simulink model "quad_dynamics"  (R2026a)
settings: Solver=ode4  StopTime=50  FixedStep=0.001
InitFcn:
  | Quad_Constant
  | %Quad_Constant_Ferry
values from neighbouring files (symbols this model uses):
  Ax = 0.0    (= 0)    [Quad_Constant.m]    (also in Quad_Constant_Ferry.m = 0.1)
  Ay = 0.0    (= 0)    [Quad_Constant.m]    (also in Quad_Constant_Ferry.m = 0.1)
  Az = 0.0    (= 0)    [Quad_Constant.m]    (also in Quad_Constant_Ferry.m = 0.1)
  b = cT_rpm * rpm_to_rads_factor    (= 1.35552545536e-05)    [Quad_Constant.m]    (also in Quad_Constant_Ferry.m = 1.144e-08)
  d = cM_rpm * rpm_to_rads_factor    (= 2.66728015938e-07)    [Quad_Constant.m]    (also in Quad_Constant_Ferry.m = 9.94e-10)
  g = 9.8100    (= 9.81)    [Quad_Constant.m]    (also in Quad_Constant_Ferry.m)
  Ixx = 0.0095    [Quad_Constant.m]    (also in Quad_Constant_Ferry.m = 0.005)
  Iyy = 0.0095    [Quad_Constant.m]    (also in Quad_Constant_Ferry.m = 0.005)
  Izz = 0.0186    [Quad_Constant.m]    (also in Quad_Constant_Ferry.m = 0.01)
  Jr = 6.5e-07    [Quad_Constant.m]    (also in Quad_Constant_Ferry.m)
  l = 0.2223    [Quad_Constant.m]    (also in Quad_Constant_Ferry.m = 0.225)
  m = 1.0230    (= 1.023)    [Quad_Constant.m]    (also in Quad_Constant_Ferry.m = 0.284)
undefined symbols (not defined in the file or in its folder): fractalcoef
libraries: mspsensorlib x1
settings Model: Creator=Umesh  LastModifiedBy=choudharyumesh

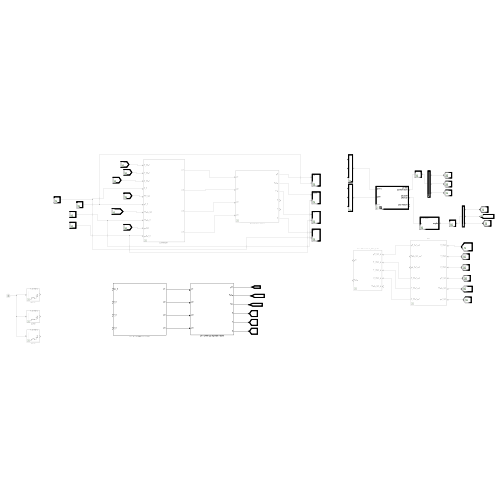
[thumbnail: Simulink's stored preview of the top-level diagram]
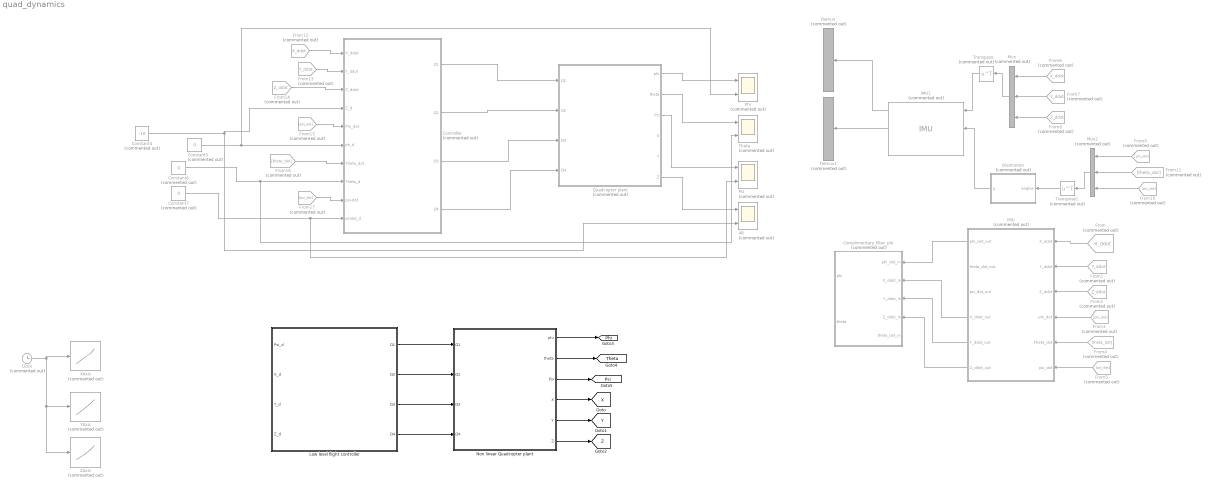
== system quad_dynamics ==
  Alt : Scope  Commented=on  NumInputPorts=2
      settings: ActiveDisplayYMinimum=-11.368140243902438  ActiveDisplayYMaximum=1.75685975609756
  Clock : Clock  Commented=on
  Complimentary_filter_phi : Subsystem  Commented=on
  Constant4 : Constant  Commented=on  Value=-10
  Constant5 : Constant  Commented=on  Value=0
  Constant6 : Constant  Commented=on  Value=0
  Constant7 : Constant  Commented=on  Value=0
  "Controller " : Subsystem  Commented=on
  Demux : Demux  Commented=on  Outputs=3
  Demux1 : Demux  Commented=on  Outputs=3
  From : From  Commented=on  GotoTag=X_ddot  TagVisibility=global
  From1 : From  Commented=on  GotoTag=Y_ddot  TagVisibility=global
  From10 : From  Commented=on  GotoTag=psi_dot  TagVisibility=global
  From11 : From  Commented=on  GotoTag=theta_dot  TagVisibility=global
  From12 : From  Commented=on  GotoTag=X_ddot  TagVisibility=global
  From13 : From  Commented=on  GotoTag=Y_ddot  TagVisibility=global
  From14 : From  Commented=on  GotoTag=Z_ddot  TagVisibility=global
  From15 : From  Commented=on  GotoTag=phi_dot  TagVisibility=global
  From16 : From  Commented=on  GotoTag=theta_dot  TagVisibility=global
  From17 : From  Commented=on  GotoTag=psi_dot  TagVisibility=global
  From2 : From  Commented=on  GotoTag=Z_ddot  TagVisibility=global
  From3 : From  Commented=on  GotoTag=phi_dot  TagVisibility=global
  From4 : From  Commented=on  GotoTag=theta_dot  TagVisibility=global
  From5 : From  Commented=on  GotoTag=psi_dot  TagVisibility=global
  From6 : From  Commented=on  GotoTag=X_ddot  TagVisibility=global
  From7 : From  Commented=on  GotoTag=Y_ddot  TagVisibility=global
  From8 : From  Commented=on  GotoTag=Z_ddot  TagVisibility=global
  From9 : From  Commented=on  GotoTag=phi_dot  TagVisibility=global
  IMU : Subsystem  Commented=on
  IMU1 : mspsensorlib/IMU  Commented=on  DispRefFrame=NED  TemperaturePort=off  Temperature=25  MagneticFieldPort=off  MagneticFieldNED=[ 27.5550, -2.4169, -16.0849 ]  MagneticFieldENU=[ -2.4169, 27.5550, 16.0849 ]  SeedDouble=67  SimulateUsing=Interpreted execution  AccelParamsMeasurementRange=Inf  AccelParamsResolution=0  AccelParamsConstantBias=[-2.755e-5, 1.565e-5, -9.942e-5]  AccelParamsAxesMisalignment=[ 100, 0, 0; 0, 100, 0; 0, 0, 100 ]  AccelParamsNoiseDensity=[ 0, 0, 0 ]  AccelParamsBiasInstability=[ 0, 0, 0 ]  AccelParamsBiasInstabilityNumerator=fractalcoef().Numerator  AccelParamsBiasInstabilityDenominator=fractalcoef().Denominator  AccelParamsRandomWalk=[ 0, 0, 0 ]  AccelParamsNoiseType=double-sided  AccelParamsTemperatureBias=[ 0, 0, 0 ]  AccelParamsTemperatureScaleFactor=[ 0, 0, 0 ]  GyroParamsMeasurementRange=Inf  GyroParamsResolution=0  GyroParamsConstantBias=[0.2001e-3, 0.2002e-3, 0.2004e-3]  GyroParamsAxesMisalignment=[ 100, 0, 0; 0, 100, 0; 0, 0, 100 ]  GyroParamsAccelerationBias=[ 0, 0, 0 ]  GyroParamsNoiseDensity=[ 0, 0, 0 ]  GyroParamsBiasInstability=[ 0, 0, 0 ]  GyroParamsBiasInstabilityNumerator=fractalcoef().Numerator  GyroParamsBiasInstabilityDenominator=fractalcoef().Denominator  GyroParamsRandomWalk=[ 0, 0, 0 ]  GyroParamsNoiseType=double-sided  GyroParamsTemperatureBias=[ 0, 0, 0 ]  GyroParamsTemperatureScaleFactor=[ 0, 0, 0 ]  MagParamsMeasurementRange=Inf  MagParamsResolution=0  MagParamsConstantBias=[-0.3223e-5, -0.1280e-5, 0.1589e-5]  MagParamsAxesMisalignment=[ 100, 0, 0; 0, 100, 0; 0, 0, 100 ]  MagParamsNoiseDensity=[ 0, 0, 0 ]  MagParamsBiasInstability=[ 0, 0, 0 ]  MagParamsBiasInstabilityNumerator=fractalcoef().Numerator  MagParamsBiasInstabilityDenominator=fractalcoef().Denominator  MagParamsRandomWalk=[ 0, 0, 0 ]  MagParamsNoiseType=double-sided  MagParamsTemperatureBias=[ 0, 0, 0 ]  MagParamsTemperatureScaleFactor=[ 0, 0, 0 ]
  Low level flight controller : Subsystem
  Mux : Mux  Commented=on  Inputs=3
  Mux2 : Mux  Commented=on  Inputs=3
  Non linear Quadcopter plant : Subsystem
  Oreintation : MATLAB Function  Commented=on  TreatAsAtomicUnit=on
  Phi : Scope  Commented=on  NumInputPorts=2
      settings: ActiveDisplayYMinimum=-5.7658911529616628  ActiveDisplayYMaximum=1.4877959493201969  DataLoggingVariableName=ScopeData2
  Psi : Scope  Commented=on  NumInputPorts=2
      settings: ActiveDisplayYMinimum=-3.9264406284982103  ActiveDisplayYMaximum=3.92682926955981
  Quadcopter plant : Subsystem  Commented=on
  Theta : Scope  Commented=on  NumInputPorts=2
      settings: ActiveDisplayYMinimum=-5.4636541903665821  ActiveDisplayYMaximum=1.4446192403780447  DataLoggingVariableName=ScopeData3
  Transpose : Math  Commented=on  Operator=transpose
  Transpose1 : Math  Commented=on  Operator=transpose
  XAxis : Lookup_n-D  Commented=on  NumberOfTableDimensions=1  BreakpointsForDimension1=[0, 5, 10, 15, 20, 25, 30]  Table=[0, 10, 0, -10, 0, 10, 0]  InterpMethod=Flat  InternalRulePriority=Speed  RndMeth=Simplest
  YAxis : Lookup_n-D  Commented=on  NumberOfTableDimensions=1  BreakpointsForDimension1=[0, 5, 10, 15, 20, 25, 30]  Table=[0, 0, 10, 0, -10, 0, 0]  InterpMethod=Flat  InternalRulePriority=Speed  RndMeth=Simplest
  ZAxis : Lookup_n-D  Commented=on  NumberOfTableDimensions=1  BreakpointsForDimension1=[0, 5, 10, 15, 20, 25, 30]  Table=[-3, -3, -3, -3, -3, -3, -3]  InterpMethod=Flat  InternalRulePriority=Speed  RndMeth=Simplest
  tag scope: Phi=global, Psi=global, Theta=global, X=global, Y=global, Z=global
  wires:
  From/1 -> IMU/1(X_ddot)
  From1/1 -> IMU/2(Y_ddot)
  From2/1 -> IMU/3(Z_ddot)
  From3/1 -> IMU/4(phi_dot)
  From4/1 -> IMU/5(Theta_dot)
  From5/1 -> IMU/6(psi_dot)
  IMU/1(phi_dot_out) -> Complimentary_filter_phi/1(phi_dot_in)
  IMU/4(X_ddot_out) -> Complimentary_filter_phi/2(X_ddot_in)
  IMU/5(Y_ddot_out) -> Complimentary_filter_phi/3(Y_ddot_in)
  IMU/6(Z_ddot_out) -> Complimentary_filter_phi/4(Z_ddot_in)
  From6/1 -> Mux/1
  From7/1 -> Mux/2
  From8/1 -> Mux/3
  Mux/1 -> Transpose/1
  From9/1 -> Mux2/1
  From10/1 -> Mux2/3
  From11/1 -> Mux2/2
  Mux2/1 -> Transpose1/1
  "Controller "/1(Ω1) -> Quadcopter plant/1(Ω1)
  "Controller "/2(Ω2) -> Quadcopter plant/2(Ω2)
  "Controller "/3(Ω3) -> Quadcopter plant/3(Ω3)
  "Controller "/4(Ω4) -> Quadcopter plant/4(Ω4)
  IMU1/2 -> Demux1/1
  IMU1/1 -> Demux/1
  Transpose/1 -> IMU1/1
  Transpose1/1 -> Oreintation/1(angles)
  Oreintation/1(q) -> IMU1/2
  From17/1 -> "Controller "/9(psi-dot)
  From16/1 -> "Controller "/7(Theta_dot)
  From15/1 -> "Controller "/5(Phi_dot)
  From12/1 -> "Controller "/1(X_ddot)
  From13/1 -> "Controller "/2(Y_ddot)
  From14/1 -> "Controller "/3(Z_ddot)
  Constant4/1 -> "Controller "/4(Z_d), Alt/2
  Constant5/1 -> Phi/2, "Controller "/6(ph_d)
  Constant6/1 -> Theta/2, "Controller "/8(Theta_d)
  Constant7/1 -> Psi/2, "Controller "/10(psidot_d)
  Quadcopter plant/6(Z) -> Alt/1
  Quadcopter plant/1(phi) -> Phi/1
  Quadcopter plant/2(theta) -> Theta/1
  Quadcopter plant/3(Psi) -> Psi/1
  Non linear Quadcopter plant/2(theta) -> [Theta]
  Non linear Quadcopter plant/3(Psi) -> [Psi]
  Non linear Quadcopter plant/4(X) -> [X]
  Non linear Quadcopter plant/5(Y) -> [Y]
  Non linear Quadcopter plant/6(Z) -> [Z]
  Low level flight controller/1(Ω1) -> Non linear Quadcopter plant/1(Ω1)
  Low level flight controller/2(Ω2) -> Non linear Quadcopter plant/2(Ω2)
  Low level flight controller/3(Ω3) -> Non linear Quadcopter plant/3(Ω3)
  Low level flight controller/4(Ω4) -> Non linear Quadcopter plant/4(Ω4)
  Clock/1 -> ZAxis/1, YAxis/1, XAxis/1
  Non linear Quadcopter plant/1(phi) -> [Phi]

== system quad_dynamics/Complimentary_filter_phi ==
  phi_dot_in : Inport
  X_ddot_in : Inport  Port=2
  Y_ddot_in : Inport  Port=3
  Z_ddot_in : Inport  Port=4
  theta_dot_in : Inport  Port=5
  High pass filter : TransferFcn  Numerator=[2 0]  Denominator=[2 1]
  High pass filter1 : TransferFcn  Numerator=[2 0]  Denominator=[2 1]
  Integrator : Integrator
  Integrator1 : Integrator
  Low pass filter : TransferFcn  Denominator=[2 1]
  MATLAB Function : MATLAB Function  TreatAsAtomicUnit=on
  Sum : Sum
  Sum1 : Sum
  phi : Outport
  theta : Outport  Port=2
  wires:
  X_ddot_in/1 -> MATLAB Function/1(X_ddot_in)
  Y_ddot_in/1 -> MATLAB Function/2(Y_ddot_in)
  Z_ddot_in/1 -> MATLAB Function/3(Z_ddot_in)
  MATLAB Function/1(Phi) -> Low pass filter/1
  phi_dot_in/1 -> Integrator/1
  Integrator/1 -> High pass filter/1
  Low pass filter/1 -> Sum/1
  High pass filter/1 -> Sum/2
  Sum/1 -> phi/1
  theta_dot_in/1 -> Integrator1/1
  Integrator1/1 -> High pass filter1/1
  High pass filter1/1 -> Sum1/2
  MATLAB Function/2(Theta) -> Sum1/1
  Sum1/1 -> theta/1

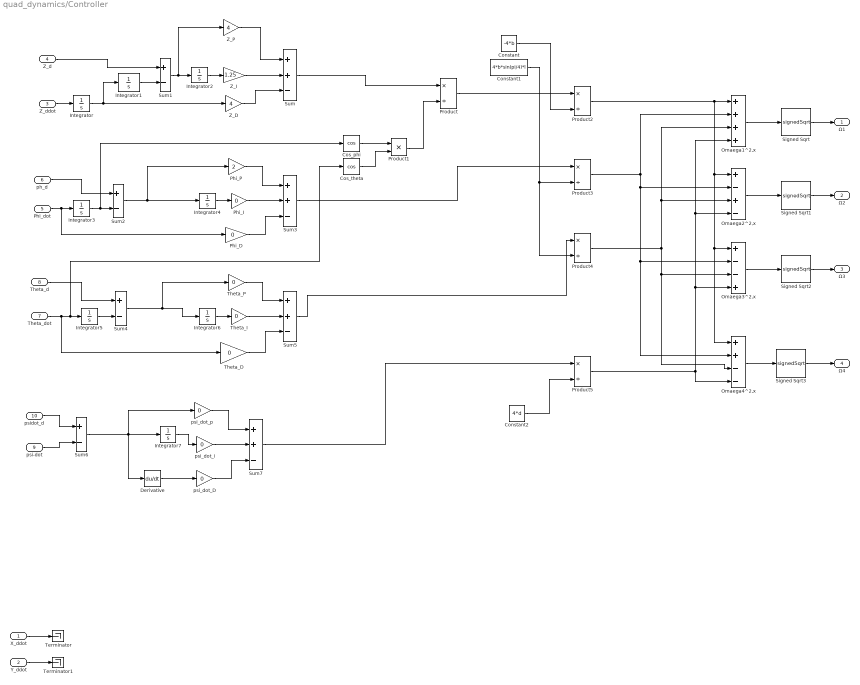
== system quad_dynamics/Controller  ==
  X_ddot : Inport
  Y_ddot : Inport  Port=2
  Z_ddot : Inport  Port=3
  Z_d : Inport  Port=4
  Phi_dot : Inport  Port=5
  ph_d : Inport  Port=6
  Theta_dot : Inport  Port=7
  Theta_d : Inport  Port=8
  psi-dot : Inport  Port=9
  psidot_d : Inport  Port=10
  Constant : Constant  Value=-4*b
  Constant1 : Constant  Value=4*b*sin(pi/4)*l
  Constant2 : Constant  Value=4*d
  Cos_phi : Trigonometry  Operator=cos
  Cos_theta : Trigonometry  Operator=cos
  Derivative : Derivative
  Integrator{,4,6..7} (4 alike) : Integrator
  Integrator1 : Integrator  UpperSaturationLimit=pi  LowerSaturationLimit=-pi
  Integrator2 : Integrator  LimitOutput=on  UpperSaturationLimit=5  LowerSaturationLimit=-5
  Integrator3 : Integrator  UpperSaturationLimit=pi  LowerSaturationLimit=-pi  WrapState=on
  Integrator5 : Integrator  UpperSaturationLimit=pi  LowerSaturationLimit=-pi  WrapState=on
  Omaega1^2,x : Sum  Inputs=++++
  Omaega2^2,x : Sum  Inputs=+-+-
  Omaega3^2,x : Sum  Inputs=+--+
  Omaega4^2,x : Sum  Inputs=++--
  Phi_D : Gain  Gain=0
  Phi_I : Gain  Gain=0
  Phi_P : Gain  Gain=2
  Product{,2..5} (5 alike) : Product  Inputs=*/
  Product1 : Product
  Signed Sqrt{,1..3} (4 alike) : Sqrt  Operator=signedSqrt
  Sum{,3,5,7} (4 alike) : Sum  Inputs=++-
  Sum{1..2,4,6} (4 alike) : Sum  Inputs=+-
  Terminator : Terminator
  Terminator1 : Terminator
  Theta_D : Gain  Gain=0
  Theta_I : Gain  Gain=0
  Theta_P : Gain  Gain=0
  Z_D : Gain  Gain=4
  Z_I : Gain  Gain=1.25
  Z_P : Gain  Gain=4
  psi_dot_D : Gain  Gain=0
  psi_dot_i : Gain  Gain=0
  psi_dot_p : Gain  Gain=0
  Ω1 : Outport
  Ω2 : Outport  Port=2
  Ω3 : Outport  Port=3
  Ω4 : Outport  Port=4
  wires:
  Z_ddot/1 -> Integrator/1
  Integrator/1 -> Z_D/1, Integrator1/1
  Integrator1/1 -> Sum1/2
  Z_d/1 -> Sum1/1
  Z_D/1 -> Sum/3
  Integrator2/1 -> Z_I/1
  Z_I/1 -> Sum/2
  Z_P/1 -> Sum/1
  Sum1/1 -> Z_P/1, Integrator2/1
  Phi_dot/1 -> Phi_D/1, Integrator3/1
  Integrator3/1 -> Cos_phi/1, Sum2/2
  ph_d/1 -> Sum2/1
  Phi_D/1 -> Sum3/3
  Integrator4/1 -> Phi_I/1
  Sum2/1 -> Phi_P/1, Integrator4/1
  Phi_I/1 -> Sum3/2
  Phi_P/1 -> Sum3/1
  Integrator5/1 -> Sum4/2
  Theta_d/1 -> Sum4/1
  Theta_P/1 -> Sum5/1
  Theta_dot/1 -> Theta_D/1, Cos_theta/1, Integrator5/1
  Theta_D/1 -> Sum5/3
  Theta_I/1 -> Sum5/2
  Integrator6/1 -> Theta_I/1
  Sum4/1 -> Theta_P/1, Integrator6/1
  psidot_d/1 -> Sum6/1
  psi_dot_i/1 -> Sum7/2
  Integrator7/1 -> psi_dot_i/1
  psi_dot_D/1 -> Sum7/3
  psi_dot_p/1 -> Sum7/1
  Sum6/1 -> Derivative/1, Integrator7/1, psi_dot_p/1
  Derivative/1 -> psi_dot_D/1
  Sum/1 -> Product/1
  Cos_phi/1 -> Product1/1
  Cos_theta/1 -> Product1/2
  Product1/1 -> Product/2
  Product/1 -> Product2/1
  Constant/1 -> Product2/2
  Constant1/1 -> Product4/2, Product3/2
  Sum3/1 -> Product3/1
  Sum5/1 -> Product4/1
  Sum7/1 -> Product5/1
  Constant2/1 -> Product5/2
  Omaega1^2,x/1 -> Signed Sqrt/1
  Signed Sqrt/1 -> Ω1/1
  Product2/1 -> Omaega4^2,x/1, Omaega3^2,x/1, Omaega2^2,x/1, Omaega1^2,x/1
  Product3/1 -> Omaega4^2,x/2, Omaega3^2,x/2, Omaega2^2,x/2, Omaega1^2,x/2
  Product4/1 -> Omaega3^2,x/3, Omaega4^2,x/3, Omaega2^2,x/3, Omaega1^2,x/3
  Product5/1 -> Omaega3^2,x/4, Omaega2^2,x/4, Omaega1^2,x/4, Omaega4^2,x/4
  Omaega2^2,x/1 -> Signed Sqrt1/1
  Signed Sqrt1/1 -> Ω2/1
  Omaega3^2,x/1 -> Signed Sqrt2/1
  Signed Sqrt2/1 -> Ω3/1
  Omaega4^2,x/1 -> Signed Sqrt3/1
  Signed Sqrt3/1 -> Ω4/1
  X_ddot/1 -> Terminator/1
  Y_ddot/1 -> Terminator1/1
  psi-dot/1 -> Sum6/2

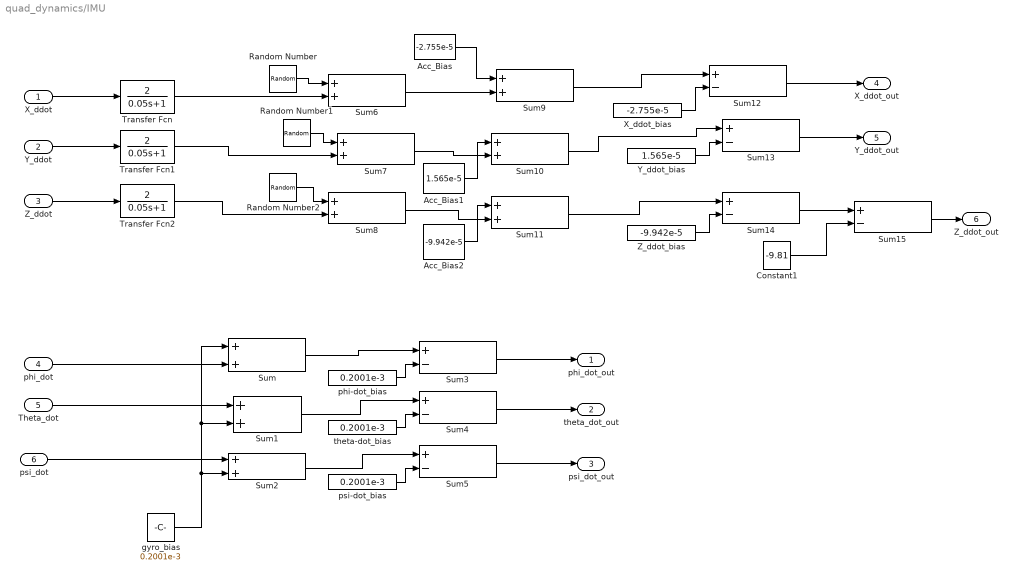
== system quad_dynamics/IMU ==
  X_ddot : Inport
  Y_ddot : Inport  Port=2
  Z_ddot : Inport  Port=3
  phi_dot : Inport  Port=4
  Theta_dot : Inport  Port=5
  psi_dot : Inport  Port=6
  Acc_Bias : Constant  Value=-2.755e-5
  Acc_Bias1 : Constant  Value=1.565e-5
  Acc_Bias2 : Constant  Value=-9.942e-5
  Constant1 : Constant  Value=-9.81
  Random Number : RandomNumber  Variance=0  Seed=1  SampleTime=0.01
  Random Number1 : RandomNumber  Variance=0  Seed=1  SampleTime=0.01
  Random Number2 : RandomNumber  Variance=0  Seed=1  SampleTime=0.01
  Sum{,1..2,6..11} (9 alike) : Sum
  Sum{3..5,12..15} (7 alike) : Sum  Inputs=+-
  Transfer Fcn : TransferFcn  Numerator=[2]  Denominator=[0.05 1]
  Transfer Fcn1 : TransferFcn  Numerator=[2]  Denominator=[0.05 1]
  Transfer Fcn2 : TransferFcn  Numerator=[2]  Denominator=[0.05 1]
  X_ddot_bias : Constant  Value=-2.755e-5
  Y_ddot_bias : Constant  Value=1.565e-5
  Z_ddot_bias : Constant  Value=-9.942e-5
  gyro_bias : Constant  Value=0.2001e-3
  phi-dot_bias : Constant  Value=0.2001e-3
  psi-dot_bias : Constant  Value=0.2001e-3
  theta-dot_bias : Constant  Value=0.2001e-3
  phi_dot_out : Outport
  theta_dot_out : Outport  Port=2
  psi_dot_out : Outport  Port=3
  X_ddot_out : Outport  Port=4
  Y_ddot_out : Outport  Port=5
  Z_ddot_out : Outport  Port=6
  wires:
  gyro_bias/1 -> Sum/1, Sum1/2, Sum2/2
  phi_dot/1 -> Sum/2
  Theta_dot/1 -> Sum1/1
  psi_dot/1 -> Sum2/1
  Sum/1 -> Sum3/1
  Sum1/1 -> Sum4/1
  Sum2/1 -> Sum5/1
  phi-dot_bias/1 -> Sum3/2
  theta-dot_bias/1 -> Sum4/2
  psi-dot_bias/1 -> Sum5/2
  Sum3/1 -> phi_dot_out/1
  Sum4/1 -> theta_dot_out/1
  Sum5/1 -> psi_dot_out/1
  Random Number2/1 -> Sum8/1
  Random Number1/1 -> Sum7/1
  Random Number/1 -> Sum6/1
  Sum6/1 -> Sum9/2
  Sum7/1 -> Sum10/2
  Sum8/1 -> Sum11/2
  Acc_Bias/1 -> Sum9/1
  Sum9/1 -> Sum12/1
  X_ddot_bias/1 -> Sum12/2
  Y_ddot_bias/1 -> Sum13/2
  Z_ddot_bias/1 -> Sum14/2
  Sum10/1 -> Sum13/1
  Sum11/1 -> Sum14/1
  Sum14/1 -> Sum15/1
  Constant1/1 -> Sum15/2
  Sum15/1 -> Z_ddot_out/1
  Sum13/1 -> Y_ddot_out/1
  Sum12/1 -> X_ddot_out/1
  X_ddot/1 -> Transfer Fcn/1
  Transfer Fcn/1 -> Sum6/2
  Y_ddot/1 -> Transfer Fcn1/1
  Z_ddot/1 -> Transfer Fcn2/1
  Transfer Fcn1/1 -> Sum7/2
  Transfer Fcn2/1 -> Sum8/2
  Acc_Bias1/1 -> Sum10/1
  Acc_Bias2/1 -> Sum11/1

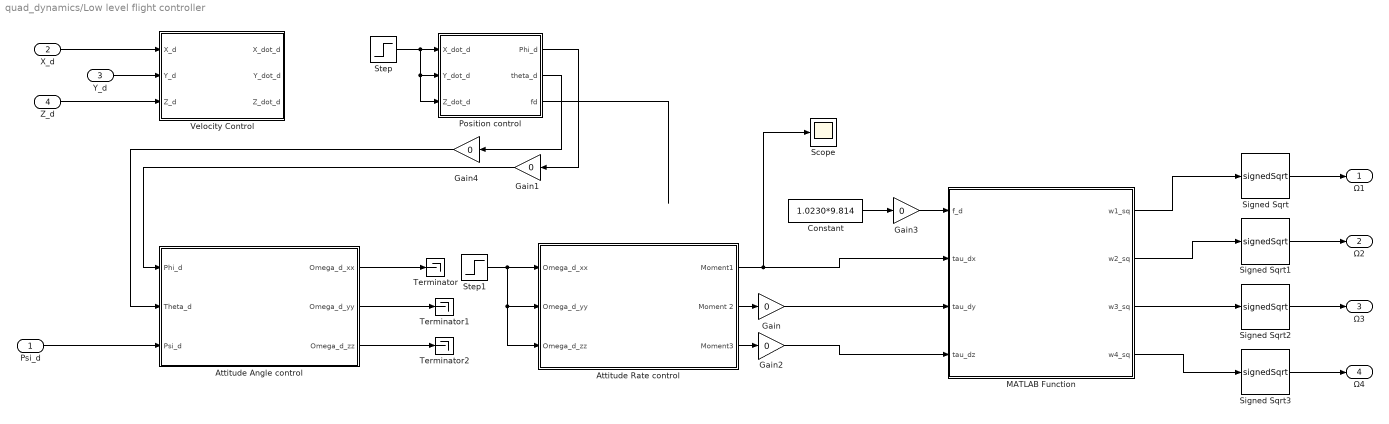
== system quad_dynamics/Low level flight controller ==
  Psi_d : Inport
  X_d : Inport  Port=2
  Y_d : Inport  Port=3
  Z_d : Inport  Port=4
  " Velocity Control" : Subsystem
  Attitude Angle control : Subsystem
  Attitude Rate control : Subsystem
  Constant : Constant  Value=1.0230*9.814
  Gain{,1..4} (5 alike) : Gain  Gain=0
  MATLAB Function : MATLAB Function  TreatAsAtomicUnit=on
  Position control : Subsystem
  Scope : Scope
      settings: ActiveDisplayYMinimum=-7.1765651912909775E+48  ActiveDisplayYMaximum=7.97396132365664E+47  DataLoggingVariableName=ScopeData11
  Signed Sqrt{,1..3} (4 alike) : Sqrt  Operator=signedSqrt
  Step : Step  FinalValue=5  SampleTime=0
  Step1 : Step  FinalValue=0.314  SampleTime=0
  Terminator : Terminator
  Terminator1 : Terminator
  Terminator2 : Terminator
  Ω1 : Outport
  Ω2 : Outport  Port=2
  Ω3 : Outport  Port=3
  Ω4 : Outport  Port=4
  wires:
  Z_d/1 -> " Velocity Control"/3(Z_d)
  Y_d/1 -> " Velocity Control"/2(Y_d)
  X_d/1 -> " Velocity Control"/1(X_d)
  Signed Sqrt1/1 -> Ω2/1
  Signed Sqrt3/1 -> Ω4/1
  Signed Sqrt/1 -> Ω1/1
  Signed Sqrt2/1 -> Ω3/1
  MATLAB Function/1(w1_sq) -> Signed Sqrt/1
  MATLAB Function/2(w2_sq) -> Signed Sqrt1/1
  MATLAB Function/3(w3_sq) -> Signed Sqrt2/1
  MATLAB Function/4(w4_sq) -> Signed Sqrt3/1
  Position control/3(fd) -> ?
  Attitude Rate control/1(Moment1) -> Scope/1, MATLAB Function/2(tau_dx)
  Attitude Rate control/2(Moment 2) -> Gain/1
  Attitude Angle control/3(Omega_d_zz) -> Terminator2/1
  Attitude Rate control/3(Moment3) -> Gain2/1
  Attitude Angle control/2(Omega_d_yy) -> Terminator1/1
  Position control/2(theta_d) -> Gain4/1
  Position control/1(Phi_d) -> Gain1/1
  Psi_d/1 -> Attitude Angle control/3(Psi_d)
  Attitude Angle control/1(Omega_d_xx) -> Terminator/1
  Gain4/1 -> Attitude Angle control/2(Theta_d)
  Step/1 -> Position control/3(Z_dot_d), Position control/2(Y_dot_d), Position control/1(X_dot_d)
  Gain1/1 -> Attitude Angle control/1(Phi_d)
  Step1/1 -> Attitude Rate control/3(Omega_d_zz), Attitude Rate control/2(Omega_d_yy), Attitude Rate control/1(Omega_d_xx)
  Gain/1 -> MATLAB Function/3(tau_dy)
  Gain2/1 -> MATLAB Function/4(tau_dz)
  Constant/1 -> Gain3/1
  Gain3/1 -> MATLAB Function/1(f_d)

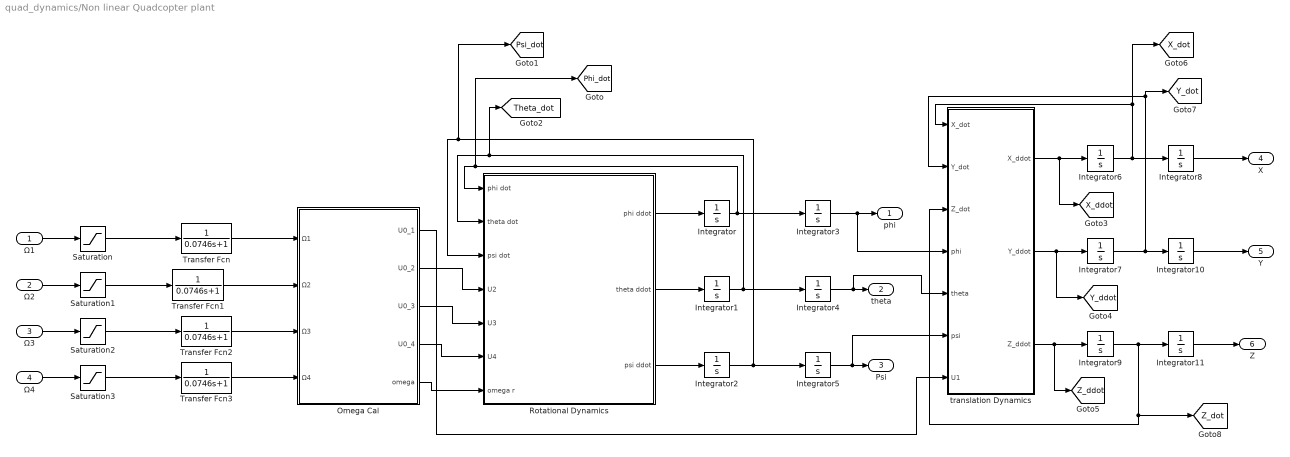
== system quad_dynamics/Non linear Quadcopter plant ==
  Ω1 : Inport
  Ω2 : Inport  Port=2
  Ω3 : Inport  Port=3
  Ω4 : Inport  Port=4
  Integrator{,1,8,10} (4 alike) : Integrator
  Integrator11 : Integrator  LimitOutput=on  UpperSaturationLimit=0
  Integrator2 : Integrator  UpperSaturationLimit=90*pi/180  LowerSaturationLimit=-90*pi/180  WrapState=on
  Integrator3 : Integrator  WrapState=on
  Integrator4 : Integrator  WrapState=on
  Integrator5 : Integrator  WrapState=on
  Integrator6 : Integrator  LimitOutput=on  UpperSaturationLimit=10  LowerSaturationLimit=-10
  Integrator7 : Integrator  LimitOutput=on  UpperSaturationLimit=10  LowerSaturationLimit=-10
  Integrator9 : Integrator  LimitOutput=on  UpperSaturationLimit=10  LowerSaturationLimit=-10
  Omega Cal : Subsystem
  Rotational Dynamics : Subsystem
  Saturation{,1..3} (4 alike) : Saturate  UpperLimit=inf  LowerLimit=0
  Transfer Fcn{,1..3} (4 alike) : TransferFcn  Denominator=[0.0746 1]
  translation Dynamics : Subsystem
  phi : Outport
  theta : Outport  Port=2
  Psi : Outport  Port=3
  X : Outport  Port=4
  Y : Outport  Port=5
  Z : Outport  Port=6
  tag scope: Phi_dot=global, Psi_dot=global, Theta_dot=global, X_ddot=global, X_dot=global, Y_ddot=global, Y_dot=global, Z_ddot=global, Z_dot=global
  wires:
  Ω1/1 -> Saturation/1
  Ω2/1 -> Saturation1/1
  Ω3/1 -> Saturation2/1
  Ω4/1 -> Saturation3/1
  Omega Cal/2(U0_2) -> Rotational Dynamics/4(" U2")
  Omega Cal/3(U0_3) -> Rotational Dynamics/5(U3)
  Omega Cal/4(U0_4) -> Rotational Dynamics/6(U4)
  Omega Cal/5(omega) -> Rotational Dynamics/7(" omega r")
  Rotational Dynamics/1(phi ddot) -> Integrator/1
  Rotational Dynamics/2(theta ddot) -> Integrator1/1
  Rotational Dynamics/3(psi ddot) -> Integrator2/1
  Integrator/1 -> Integrator3/1, [Phi_dot], Rotational Dynamics/1(phi dot)
  Integrator1/1 -> Integrator4/1, [Theta_dot], Rotational Dynamics/2(theta dot)
  Integrator2/1 -> [Psi_dot], Rotational Dynamics/3(psi dot), Integrator5/1
  Integrator3/1 -> translation Dynamics/4(phi), phi/1
  Integrator4/1 -> translation Dynamics/5(theta), theta/1
  Integrator5/1 -> translation Dynamics/6(psi), Psi/1
  translation Dynamics/1(X_ddot) -> [X_ddot], Integrator6/1
  translation Dynamics/2(Y_ddot) -> Integrator7/1, [Y_ddot]
  translation Dynamics/3(Z_ddot) -> Integrator9/1, [Z_ddot]
  Integrator9/1 -> [Z_dot], translation Dynamics/3(Z_dot), Integrator11/1
  Integrator7/1 -> [Y_dot], translation Dynamics/2(Y_dot), Integrator10/1
  Integrator6/1 -> [X_dot], translation Dynamics/1(X_dot), Integrator8/1
  Omega Cal/1(U0_1) -> translation Dynamics/7(U1)
  Integrator8/1 -> X/1
  Integrator10/1 -> Y/1
  Integrator11/1 -> Z/1
  Saturation/1 -> Transfer Fcn/1
  Saturation1/1 -> Transfer Fcn1/1
  Saturation2/1 -> Transfer Fcn2/1
  Saturation3/1 -> Transfer Fcn3/1
  Transfer Fcn/1 -> Omega Cal/1(Ω1)
  Transfer Fcn1/1 -> Omega Cal/2(Ω2)
  Transfer Fcn2/1 -> Omega Cal/3(Ω3)
  Transfer Fcn3/1 -> Omega Cal/4(Ω4)

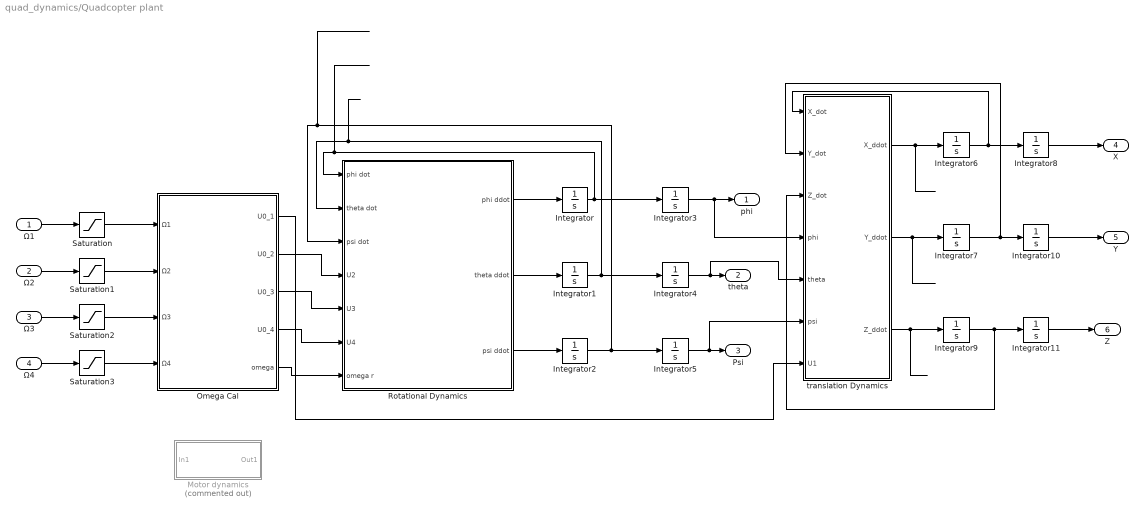
== system quad_dynamics/Quadcopter plant ==
  Ω1 : Inport
  Ω2 : Inport  Port=2
  Ω3 : Inport  Port=3
  Ω4 : Inport  Port=4
  Integrator{,1,6..10} (7 alike) : Integrator
  Integrator11 : Integrator  LimitOutput=on  UpperSaturationLimit=0
  Integrator2 : Integrator  LimitOutput=on  UpperSaturationLimit=90*pi/180  LowerSaturationLimit=-90*pi/180
  Integrator3 : Integrator  WrapState=on
  Integrator4 : Integrator  WrapState=on
  Integrator5 : Integrator  WrapState=on
  Motor dynamics : Subsystem  Commented=on
  Omega Cal : Subsystem
  Rotational Dynamics : Subsystem
  Saturation{,1..3} (4 alike) : Saturate  UpperLimit=inf  LowerLimit=0
  translation Dynamics : Subsystem
  phi : Outport
  theta : Outport  Port=2
  Psi : Outport  Port=3
  X : Outport  Port=4
  Y : Outport  Port=5
  Z : Outport  Port=6
  wires:
  Ω1/1 -> Saturation/1
  Ω2/1 -> Saturation1/1
  Ω3/1 -> Saturation2/1
  Ω4/1 -> Saturation3/1
  Omega Cal/2(U0_2) -> Rotational Dynamics/4(" U2")
  Omega Cal/3(U0_3) -> Rotational Dynamics/5(U3)
  Omega Cal/4(U0_4) -> Rotational Dynamics/6(U4)
  Omega Cal/5(omega) -> Rotational Dynamics/7(" omega r")
  Rotational Dynamics/1(phi ddot) -> Integrator/1
  Rotational Dynamics/2(theta ddot) -> Integrator1/1
  Rotational Dynamics/3(psi ddot) -> Integrator2/1
  Integrator/1 -> Integrator3/1, Rotational Dynamics/1(phi dot)
  Integrator1/1 -> Integrator4/1, Rotational Dynamics/2(theta dot)
  Integrator2/1 -> Rotational Dynamics/3(psi dot), Integrator5/1
  Integrator3/1 -> translation Dynamics/4(phi), phi/1
  Integrator4/1 -> translation Dynamics/5(theta), theta/1
  Integrator5/1 -> translation Dynamics/6(psi), Psi/1
  translation Dynamics/1(X_ddot) -> Integrator6/1
  translation Dynamics/2(Y_ddot) -> Integrator7/1
  translation Dynamics/3(Z_ddot) -> Integrator9/1
  Integrator9/1 -> translation Dynamics/3(Z_dot), Integrator11/1
  Integrator7/1 -> translation Dynamics/2(Y_dot), Integrator10/1
  Integrator6/1 -> translation Dynamics/1(X_dot), Integrator8/1
  Omega Cal/1(U0_1) -> translation Dynamics/7(U1)
  Integrator8/1 -> X/1
  Integrator10/1 -> Y/1
  Integrator11/1 -> Z/1
  Saturation/1 -> Omega Cal/1(Ω1)
  Saturation1/1 -> Omega Cal/2(Ω2)
  Saturation2/1 -> Omega Cal/3(Ω3)
  Saturation3/1 -> Omega Cal/4(Ω4)

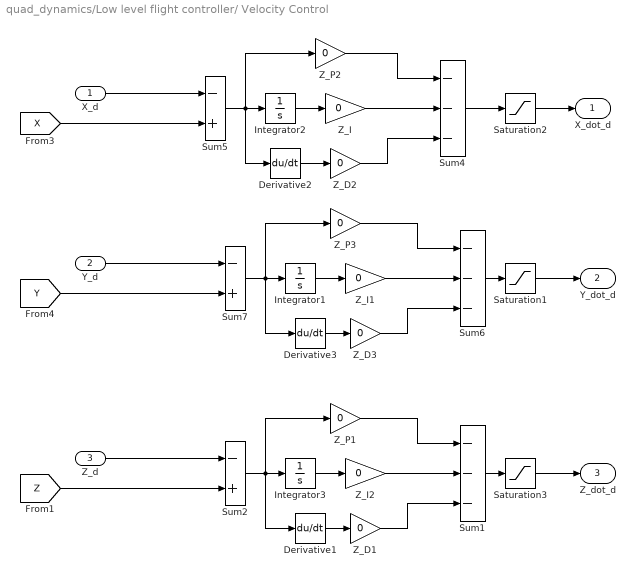
== system quad_dynamics/Low level flight controller/ Velocity Control ==
  X_d : Inport
  Y_d : Inport  Port=2
  Z_d : Inport  Port=3
  Derivative1 : Derivative
  Derivative2 : Derivative
  Derivative3 : Derivative
  Integrator1 : Integrator  LimitOutput=on  UpperSaturationLimit=5  LowerSaturationLimit=-5
  Integrator2 : Integrator  LimitOutput=on  UpperSaturationLimit=5  LowerSaturationLimit=-5
  Integrator3 : Integrator  LimitOutput=on  UpperSaturationLimit=5  LowerSaturationLimit=-5
  Saturation1 : Saturate  UpperLimit=5  LowerLimit=-5
  Saturation2 : Saturate  UpperLimit=5  LowerLimit=-5
  Saturation3 : Saturate  UpperLimit=5  LowerLimit=-5
  Sum1 : Sum  Inputs=---
  Sum2 : Sum  Inputs=-+
  Sum4 : Sum  Inputs=---
  Sum5 : Sum  Inputs=-+
  Sum6 : Sum  Inputs=---
  Sum7 : Sum  Inputs=-+
  Z_D1 : Gain  Gain=0
  Z_D2 : Gain  Gain=0
  Z_D3 : Gain  Gain=0
  Z_I : Gain  Gain=0
  Z_I1 : Gain  Gain=0
  Z_I2 : Gain  Gain=0
  Z_P1 : Gain  Gain=0
  Z_P2 : Gain  Gain=0
  Z_P3 : Gain  Gain=0
  X_dot_d : Outport
  Y_dot_d : Outport  Port=2
  Z_dot_d : Outport  Port=3
  wires:
  Saturation1/1 -> Y_dot_d/1
  Sum7/1 -> Derivative3/1, Z_P3/1, Integrator1/1
  Z_I/1 -> Sum4/2
  Integrator2/1 -> Z_I/1
  Sum4/1 -> Saturation2/1
  Sum5/1 -> Derivative2/1, Z_P2/1, Integrator2/1
  [X] -> Sum5/2
  Z_I1/1 -> Sum6/2
  [Y] -> Sum7/2
  Z_D2/1 -> Sum4/3
  Sum6/1 -> Saturation1/1
  X_d/1 -> Sum5/1
  Z_D3/1 -> Sum6/3
  Z_P3/1 -> Sum6/1
  Integrator1/1 -> Z_I1/1
  Saturation2/1 -> X_dot_d/1
  Y_d/1 -> Sum7/1
  Z_P2/1 -> Sum4/1
  Derivative3/1 -> Z_D3/1
  Derivative2/1 -> Z_D2/1
  Derivative1/1 -> Z_D1/1
  Integrator3/1 -> Z_I2/1
  Z_D1/1 -> Sum1/3
  Sum1/1 -> Saturation3/1
  Z_P1/1 -> Sum1/1
  [Z] -> Sum2/2
  Sum2/1 -> Derivative1/1, Z_P1/1, Integrator3/1
  Z_d/1 -> Sum2/1
  Saturation3/1 -> Z_dot_d/1
  Z_I2/1 -> Sum1/2

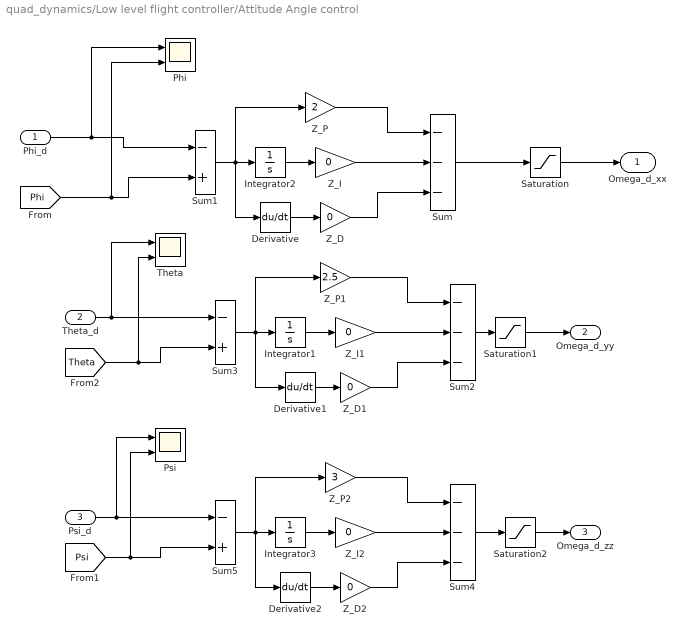
== system quad_dynamics/Low level flight controller/Attitude Angle control ==
  Phi_d : Inport
  Theta_d : Inport  Port=2
  Psi_d : Inport  Port=3
  Derivative : Derivative
  Derivative1 : Derivative
  Derivative2 : Derivative
  Integrator1 : Integrator  LimitOutput=on  UpperSaturationLimit=5  LowerSaturationLimit=-5
  Integrator2 : Integrator  LimitOutput=on  UpperSaturationLimit=5  LowerSaturationLimit=-5
  Integrator3 : Integrator  LimitOutput=on  UpperSaturationLimit=5  LowerSaturationLimit=-5
  Phi : Scope  NumInputPorts=2
      settings: ActiveDisplayYMinimum=0.47692787421581839  ActiveDisplayYMaximum=0.539888257900924  DataLoggingVariableName=ScopeData6
  Psi : Scope  NumInputPorts=2
      settings: ActiveDisplayYMinimum=-1  ActiveDisplayYMaximum=1  DataLoggingVariableName=ScopeData8
  Saturation : Saturate  UpperLimit=0.55  LowerLimit=-0.55
  Saturation1 : Saturate  UpperLimit=0.55  LowerLimit=-0.55
  Saturation2 : Saturate  UpperLimit=0.55  LowerLimit=-0.55
  Sum : Sum  Inputs=---
  Sum1 : Sum  Inputs=-+
  Sum2 : Sum  Inputs=---
  Sum3 : Sum  Inputs=-+
  Sum4 : Sum  Inputs=---
  Sum5 : Sum  Inputs=-+
  Theta : Scope  NumInputPorts=2
      settings: ActiveDisplayYMinimum=0.51668180079664749  ActiveDisplayYMaximum=0.52517851087666356  DataLoggingVariableName=ScopeData7
  Z_D : Gain  Gain=0
  Z_D1 : Gain  Gain=0
  Z_D2 : Gain  Gain=0
  Z_I : Gain  Gain=0
  Z_I1 : Gain  Gain=0
  Z_I2 : Gain  Gain=0
  Z_P : Gain  Gain=2
  Z_P1 : Gain  Gain=2.5
  Z_P2 : Gain  Gain=3
  Omega_d_xx : Outport
  Omega_d_yy : Outport  Port=2
  Omega_d_zz : Outport  Port=3
  wires:
  Sum4/1 -> Saturation2/1
  Theta_d/1 -> Theta/1, Sum3/1
  Integrator1/1 -> Z_I1/1
  Z_D1/1 -> Sum2/3
  Z_P1/1 -> Sum2/1
  Sum2/1 -> Saturation1/1
  Z_D/1 -> Sum/3
  Z_P/1 -> Sum/1
  Sum1/1 -> Derivative/1, Z_P/1, Integrator2/1
  Psi_d/1 -> Psi/1, Sum5/1
  Z_I1/1 -> Sum2/2
  Integrator2/1 -> Z_I/1
  Sum5/1 -> Derivative2/1, Z_P2/1, Integrator3/1
  Integrator3/1 -> Z_I2/1
  Z_I2/1 -> Sum4/2
  Z_D2/1 -> Sum4/3
  Z_P2/1 -> Sum4/1
  Z_I/1 -> Sum/2
  Sum3/1 -> Derivative1/1, Z_P1/1, Integrator1/1
  Saturation/1 -> Omega_d_xx/1
  Saturation1/1 -> Omega_d_yy/1
  Saturation2/1 -> Omega_d_zz/1
  Derivative/1 -> Z_D/1
  Derivative1/1 -> Z_D1/1
  Derivative2/1 -> Z_D2/1
  [Phi] -> Phi/2, Sum1/2
  Phi_d/1 -> Phi/1, Sum1/1
  [Theta] -> Theta/2, Sum3/2
  [Psi] -> Psi/2, Sum5/2
  Sum/1 -> Saturation/1

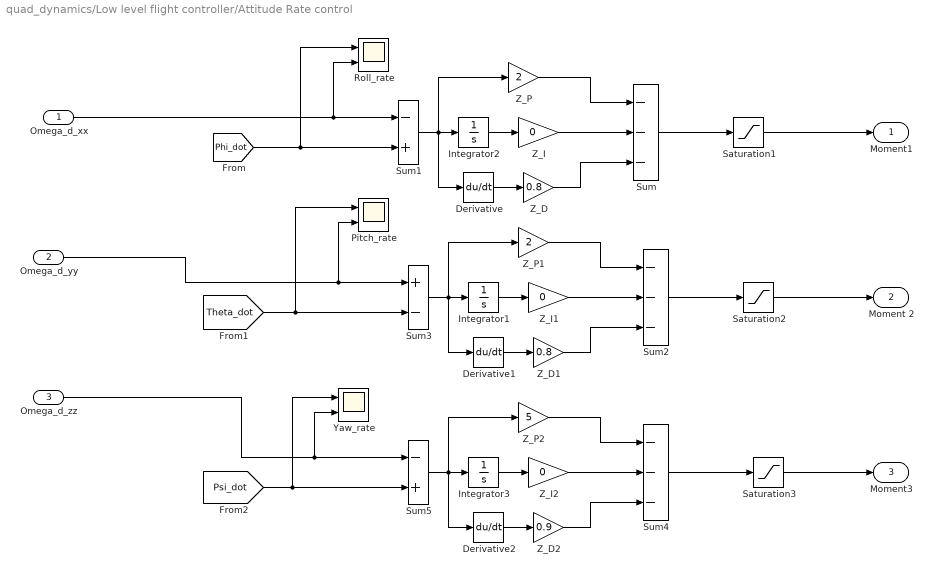
== system quad_dynamics/Low level flight controller/Attitude Rate control ==
  Omega_d_xx : Inport
  Omega_d_yy : Inport  Port=2
  Omega_d_zz : Inport  Port=3
  Derivative : Derivative
  Derivative1 : Derivative
  Derivative2 : Derivative
  Integrator1 : Integrator  LimitOutput=on  UpperSaturationLimit=5  LowerSaturationLimit=-5
  Integrator2 : Integrator  LimitOutput=on  UpperSaturationLimit=5  LowerSaturationLimit=-5
  Integrator3 : Integrator  LimitOutput=on  UpperSaturationLimit=5  LowerSaturationLimit=-5
  Pitch_rate : Scope  NumInputPorts=2
      settings: ActiveDisplayYMinimum=-0.039249999999999993  ActiveDisplayYMaximum=0.35325  DataLoggingVariableName=ScopeData5
  Roll_rate : Scope  NumInputPorts=2
      settings: ActiveDisplayYMinimum=-0.039249999999999993  ActiveDisplayYMaximum=0.35325  DataLoggingVariableName=ScopeData4
  Saturation1 : Saturate  UpperLimit=5  LowerLimit=-5
  Saturation2 : Saturate  UpperLimit=5  LowerLimit=-5
  Saturation3 : Saturate  UpperLimit=5  LowerLimit=-5
  Sum : Sum  Inputs=---
  Sum1 : Sum  Inputs=-+
  Sum2 : Sum  Inputs=---
  Sum3 : Sum  Inputs=+-
  Sum4 : Sum  Inputs=---
  Sum5 : Sum  Inputs=-+
  Yaw_rate : Scope  NumInputPorts=2
      settings: ActiveDisplayYMinimum=0.3131810994644782  ActiveDisplayYMaximum=0.31422355691852305  DataLoggingVariableName=ScopeData5
  Z_D : Gain  Gain=0.8
  Z_D1 : Gain  Gain=0.8
  Z_D2 : Gain  Gain=0.9
  Z_I : Gain  Gain=0
  Z_I1 : Gain  Gain=0
  Z_I2 : Gain  Gain=0
  Z_P : Gain  Gain=2
  Z_P1 : Gain  Gain=2
  Z_P2 : Gain  Gain=5
  Moment1 : Outport
  Moment 2 : Outport  Port=2
  Moment3 : Outport  Port=3
  wires:
  Z_I/1 -> Sum/2
  Integrator2/1 -> Z_I/1
  Sum1/1 -> Derivative/1, Z_P/1, Integrator2/1
  Z_D/1 -> Sum/3
  [Phi_dot] -> Roll_rate/1, Sum1/2
  Z_P/1 -> Sum/1
  Derivative/1 -> Z_D/1
  Derivative1/1 -> Z_D1/1
  Z_D1/1 -> Sum2/3
  Z_I1/1 -> Sum2/2
  Z_P1/1 -> Sum2/1
  [Theta_dot] -> Pitch_rate/1, Sum3/2
  Integrator1/1 -> Z_I1/1
  Sum3/1 -> Derivative1/1, Z_P1/1, Integrator1/1
  Derivative2/1 -> Z_D2/1
  Z_D2/1 -> Sum4/3
  Z_I2/1 -> Sum4/2
  Z_P2/1 -> Sum4/1
  [Psi_dot] -> Yaw_rate/1, Sum5/2
  Integrator3/1 -> Z_I2/1
  Sum5/1 -> Derivative2/1, Z_P2/1, Integrator3/1
  Sum2/1 -> Saturation2/1
  Sum4/1 -> Saturation3/1
  Omega_d_yy/1 -> Pitch_rate/2, Sum3/1
  Omega_d_zz/1 -> Yaw_rate/2, Sum5/1
  Omega_d_xx/1 -> Roll_rate/2, Sum1/1
  Sum/1 -> Saturation1/1
  Saturation1/1 -> Moment1/1
  Saturation2/1 -> Moment 2/1
  Saturation3/1 -> Moment3/1

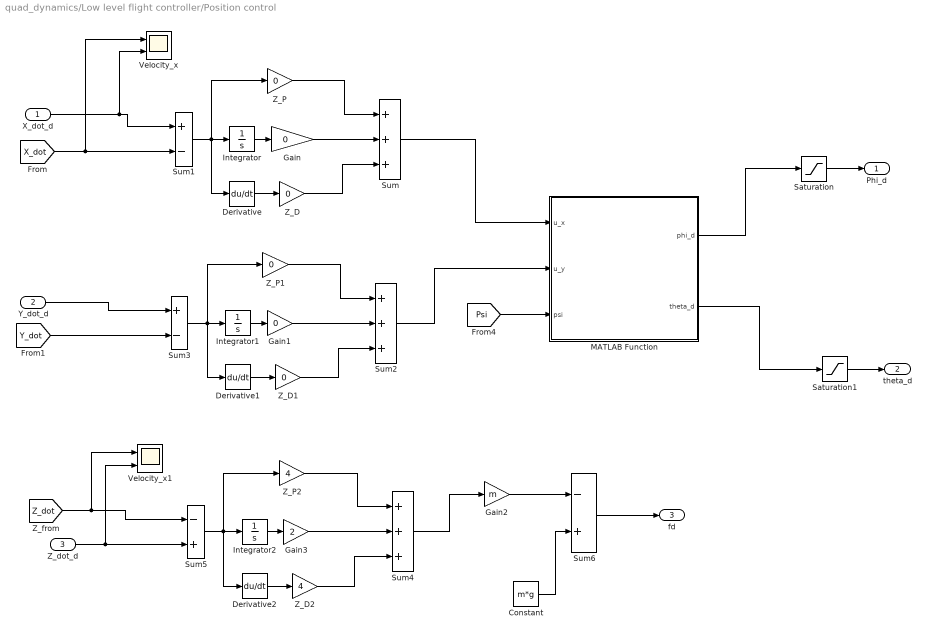
== system quad_dynamics/Low level flight controller/Position control ==
  X_dot_d : Inport
  Y_dot_d : Inport  Port=2
  Z_dot_d : Inport  Port=3
  Constant : Constant  Value=m*g
  Derivative : Derivative
  Derivative1 : Derivative
  Derivative2 : Derivative
  Gain : Gain  Gain=0
  Gain1 : Gain  Gain=0
  Gain2 : Gain  Gain=m
  Gain3 : Gain  Gain=2
  Integrator : Integrator
  Integrator1 : Integrator
  Integrator2 : Integrator
  MATLAB Function : MATLAB Function  TreatAsAtomicUnit=on
  Saturation : Saturate  UpperLimit=0.40  LowerLimit=-0.40
  Saturation1 : Saturate  UpperLimit=0.40  LowerLimit=-0.40
  Sum : Sum  Inputs=+++
  Sum1 : Sum  Inputs=+-
  Sum2 : Sum  Inputs=+++
  Sum3 : Sum  Inputs=+-
  Sum4 : Sum  Inputs=+++
  Sum5 : Sum  Inputs=-+
  Sum6 : Sum  Inputs=-+
  Velocity_x : Scope  NumInputPorts=2
      settings: ActiveDisplayYMinimum=-0.62499999999999989  ActiveDisplayYMaximum=5.625  DataLoggingVariableName=ScopeData9
  Velocity_x1 : Scope  NumInputPorts=2
      settings: ActiveDisplayYMinimum=-1.2499999999999998  ActiveDisplayYMaximum=11.25  DataLoggingVariableName=ScopeData10
  Z_D : Gain  Gain=0
  Z_D1 : Gain  Gain=0
  Z_D2 : Gain  Gain=4
  Z_P : Gain  Gain=0
  Z_P1 : Gain  Gain=0
  Z_P2 : Gain  Gain=4
  Phi_d : Outport
  theta_d : Outport  Port=2
  fd : Outport  Port=3
  wires:
  [Psi] -> MATLAB Function/3(psi)
  [X_dot] -> Velocity_x/1, Sum1/2
  Z_P/1 -> Sum/1
  Sum1/1 -> Derivative/1, Integrator/1, Z_P/1
  Derivative/1 -> Z_D/1
  MATLAB Function/2(theta_d) -> Saturation1/1
  Sum/1 -> MATLAB Function/1(u_x)
  MATLAB Function/1(phi_d) -> Saturation/1
  X_dot_d/1 -> Velocity_x/2, Sum1/1
  Z_D/1 -> Sum/3
  Gain/1 -> Sum/2
  Integrator/1 -> Gain/1
  Saturation/1 -> Phi_d/1
  Saturation1/1 -> theta_d/1
  [Y_dot] -> Sum3/2
  Z_D1/1 -> Sum2/3
  Z_P1/1 -> Sum2/1
  Gain1/1 -> Sum2/2
  Derivative1/1 -> Z_D1/1
  Integrator1/1 -> Gain1/1
  Sum3/1 -> Derivative1/1, Integrator1/1, Z_P1/1
  Sum2/1 -> MATLAB Function/2(u_y)
  Y_dot_d/1 -> Sum3/1
  Constant/1 -> Sum6/2
  Gain2/1 -> Sum6/1
  Sum6/1 -> fd/1
  [Z_dot] -> Velocity_x1/1, Sum5/1
  Z_dot_d/1 -> Velocity_x1/2, Sum5/2
  Sum5/1 -> Derivative2/1, Integrator2/1, Z_P2/1
  Gain3/1 -> Sum4/2
  Derivative2/1 -> Z_D2/1
  Z_P2/1 -> Sum4/1
  Z_D2/1 -> Sum4/3
  Integrator2/1 -> Gain3/1
  Sum4/1 -> Gain2/1

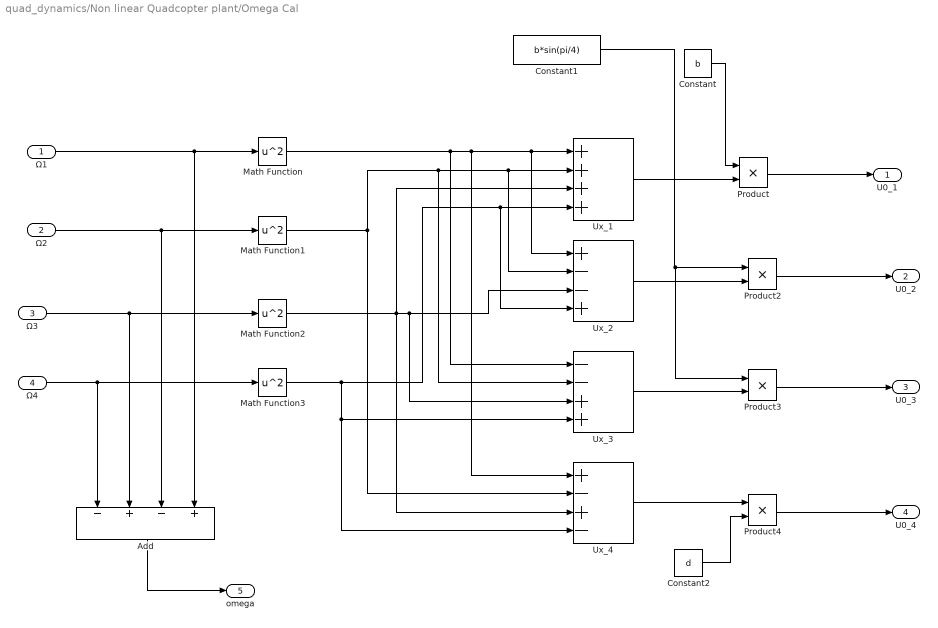
== system quad_dynamics/Non linear Quadcopter plant/Omega Cal ==
  Ω1 : Inport
  Ω2 : Inport  Port=2
  Ω3 : Inport  Port=3
  Ω4 : Inport  Port=4
  Add : Sum  Inputs=-+-+
  Constant : Constant  Value=b
  Constant1 : Constant  Value=b*sin(pi/4)
  Constant2 : Constant  Value=d
  Math Function{,1..3} (4 alike) : Math  Operator=square
  Product{,2..4} (4 alike) : Product
  Ux_1 : Sum  Inputs=++++
  Ux_2 : Sum  Inputs=+--+
  Ux_3 : Sum  Inputs=--++
  Ux_4 : Sum  Inputs=+-+-
  U0_1 : Outport
  U0_2 : Outport  Port=2
  U0_3 : Outport  Port=3
  U0_4 : Outport  Port=4
  omega : Outport  Port=5
  wires:
  Ω1/1 -> Math Function/1, Add/4
  Ω2/1 -> Math Function1/1, Add/3
  Ω3/1 -> Math Function2/1, Add/2
  Ω4/1 -> Math Function3/1, Add/1
  Add/1 -> omega/1
  Math Function/1 -> Ux_3/1, Ux_1/1, Ux_2/1, Ux_4/1
  Math Function1/1 -> Ux_4/2, Ux_3/2, Ux_2/2, Ux_1/2
  Math Function2/1 -> Ux_1/3, Ux_3/3, Ux_2/3, Ux_4/3
  Math Function3/1 -> Ux_2/4, Ux_1/4, Ux_3/4, Ux_4/4
  Constant/1 -> Product/1
  Ux_1/1 -> Product/2
  Product/1 -> U0_1/1
  Constant1/1 -> Product3/1, Product2/1
  Ux_2/1 -> Product2/2
  Ux_3/1 -> Product3/2
  Ux_4/1 -> Product4/1
  Constant2/1 -> Product4/2
  Product2/1 -> U0_2/1
  Product3/1 -> U0_3/1
  Product4/1 -> U0_4/1

== system quad_dynamics/Non linear Quadcopter plant/Rotational Dynamics ==
  phi dot : Inport
  theta dot : Inport  Port=2
  psi dot : Inport  Port=3
  " U2" : Inport  Port=4
  U3 : Inport  Port=5
  U4 : Inport  Port=6
  " omega r" : Inport  Port=7
  MATLAB Function : MATLAB Function  TreatAsAtomicUnit=on
  MATLAB Function1 : MATLAB Function  TreatAsAtomicUnit=on
  MATLAB Function2 : MATLAB Function  TreatAsAtomicUnit=on
  phi ddot : Outport
  theta ddot : Outport  Port=2
  psi ddot : Outport  Port=3
  wires:
  phi dot/1 -> MATLAB Function1/1(phi_dot), MATLAB Function2/1(phi_dot)
  theta dot/1 -> MATLAB Function/1(theta_dot), MATLAB Function2/2(theta_dot)
  psi dot/1 -> MATLAB Function/2(psi_dot), MATLAB Function1/2(psi_dot)
  " omega r"/1 -> MATLAB Function1/3(Omega_r), MATLAB Function/3(Omega_r)
  " U2"/1 -> MATLAB Function/4(U2)
  U3/1 -> MATLAB Function1/4(U3)
  U4/1 -> MATLAB Function2/3(U4)
  MATLAB Function/1(phi_ddot) -> phi ddot/1
  MATLAB Function1/1(theta_ddot) -> theta ddot/1
  MATLAB Function2/1(psi_ddot) -> psi ddot/1

== system quad_dynamics/Non linear Quadcopter plant/translation Dynamics ==
  X_dot : Inport
  Y_dot : Inport  Port=2
  Z_dot : Inport  Port=3
  phi : Inport  Port=4
  theta : Inport  Port=5
  psi : Inport  Port=6
  U1 : Inport  Port=7
  MATLAB Function : MATLAB Function  TreatAsAtomicUnit=on
  MATLAB Function1 : MATLAB Function  TreatAsAtomicUnit=on
  MATLAB Function2 : MATLAB Function  TreatAsAtomicUnit=on
  X_ddot : Outport
  Y_ddot : Outport  Port=2
  Z_ddot : Outport  Port=3
  wires:
  X_dot/1 -> MATLAB Function/4(X_dot)
  Y_dot/1 -> MATLAB Function1/4(Y_dot)
  Z_dot/1 -> MATLAB Function2/3(Z_dot)
  phi/1 -> MATLAB Function2/1(phi), MATLAB Function1/1(phi), MATLAB Function/1(phi)
  theta/1 -> MATLAB Function/2(theta), MATLAB Function1/2(theta), MATLAB Function2/2(theta)
  psi/1 -> MATLAB Function/3(psi), MATLAB Function1/3(psi)
  U1/1 -> MATLAB Function/5(U1), MATLAB Function1/5(U1), MATLAB Function2/4(U1)
  MATLAB Function/1(X_ddot) -> X_ddot/1
  MATLAB Function2/1(Z_ddot) -> Z_ddot/1
  MATLAB Function1/1(Y_ddot) -> Y_ddot/1

== system quad_dynamics/Quadcopter plant/Motor dynamics ==
  In1 : Inport
  Out1 : Outport
  wires:
  In1/1 -> Out1/1

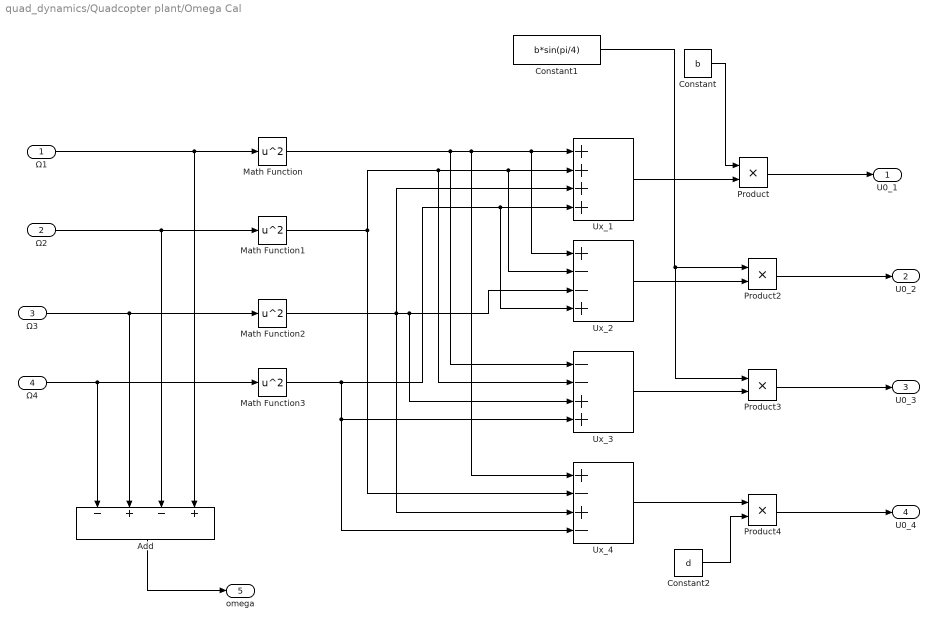
== system quad_dynamics/Quadcopter plant/Omega Cal ==
  Ω1 : Inport
  Ω2 : Inport  Port=2
  Ω3 : Inport  Port=3
  Ω4 : Inport  Port=4
  Add : Sum  Inputs=-+-+
  Constant : Constant  Value=b
  Constant1 : Constant  Value=b*sin(pi/4)
  Constant2 : Constant  Value=d
  Math Function{,1..3} (4 alike) : Math  Operator=square
  Product{,2..4} (4 alike) : Product
  Ux_1 : Sum  Inputs=++++
  Ux_2 : Sum  Inputs=+--+
  Ux_3 : Sum  Inputs=--++
  Ux_4 : Sum  Inputs=+-+-
  U0_1 : Outport
  U0_2 : Outport  Port=2
  U0_3 : Outport  Port=3
  U0_4 : Outport  Port=4
  omega : Outport  Port=5
  wires:
  Ω1/1 -> Math Function/1, Add/4
  Ω2/1 -> Math Function1/1, Add/3
  Ω3/1 -> Math Function2/1, Add/2
  Ω4/1 -> Math Function3/1, Add/1
  Add/1 -> omega/1
  Math Function/1 -> Ux_3/1, Ux_1/1, Ux_2/1, Ux_4/1
  Math Function1/1 -> Ux_4/2, Ux_3/2, Ux_2/2, Ux_1/2
  Math Function2/1 -> Ux_1/3, Ux_3/3, Ux_2/3, Ux_4/3
  Math Function3/1 -> Ux_2/4, Ux_1/4, Ux_3/4, Ux_4/4
  Constant/1 -> Product/1
  Ux_1/1 -> Product/2
  Product/1 -> U0_1/1
  Constant1/1 -> Product3/1, Product2/1
  Ux_2/1 -> Product2/2
  Ux_3/1 -> Product3/2
  Ux_4/1 -> Product4/1
  Constant2/1 -> Product4/2
  Product2/1 -> U0_2/1
  Product3/1 -> U0_3/1
  Product4/1 -> U0_4/1

== system quad_dynamics/Quadcopter plant/Rotational Dynamics ==
  phi dot : Inport
  theta dot : Inport  Port=2
  psi dot : Inport  Port=3
  " U2" : Inport  Port=4
  U3 : Inport  Port=5
  U4 : Inport  Port=6
  " omega r" : Inport  Port=7
  MATLAB Function : MATLAB Function  TreatAsAtomicUnit=on
  MATLAB Function1 : MATLAB Function  TreatAsAtomicUnit=on
  MATLAB Function2 : MATLAB Function  TreatAsAtomicUnit=on
  phi ddot : Outport
  theta ddot : Outport  Port=2
  psi ddot : Outport  Port=3
  wires:
  phi dot/1 -> MATLAB Function1/1(phi_dot), MATLAB Function2/1(phi_dot)
  theta dot/1 -> MATLAB Function/1(theta_dot), MATLAB Function2/2(theta_dot)
  psi dot/1 -> MATLAB Function/2(psi_dot), MATLAB Function1/2(psi_dot)
  " omega r"/1 -> MATLAB Function1/3(Omega_r), MATLAB Function/3(Omega_r)
  " U2"/1 -> MATLAB Function/4(U2)
  U3/1 -> MATLAB Function1/4(U3)
  U4/1 -> MATLAB Function2/3(U4)
  MATLAB Function/1(phi_ddot) -> phi ddot/1
  MATLAB Function1/1(theta_ddot) -> theta ddot/1
  MATLAB Function2/1(psi_ddot) -> psi ddot/1

== system quad_dynamics/Quadcopter plant/translation Dynamics ==
  X_dot : Inport
  Y_dot : Inport  Port=2
  Z_dot : Inport  Port=3
  phi : Inport  Port=4
  theta : Inport  Port=5
  psi : Inport  Port=6
  U1 : Inport  Port=7
  MATLAB Function : MATLAB Function  TreatAsAtomicUnit=on
  MATLAB Function1 : MATLAB Function  TreatAsAtomicUnit=on
  MATLAB Function2 : MATLAB Function  TreatAsAtomicUnit=on
  X_ddot : Outport
  Y_ddot : Outport  Port=2
  Z_ddot : Outport  Port=3
  wires:
  X_dot/1 -> MATLAB Function/4(X_dot)
  Y_dot/1 -> MATLAB Function1/4(Y_dot)
  Z_dot/1 -> MATLAB Function2/3(Z_dot)
  phi/1 -> MATLAB Function2/1(phi), MATLAB Function1/1(phi), MATLAB Function/1(phi)
  theta/1 -> MATLAB Function/2(theta), MATLAB Function1/2(theta), MATLAB Function2/2(theta)
  psi/1 -> MATLAB Function/3(psi), MATLAB Function1/3(psi)
  U1/1 -> MATLAB Function/5(U1), MATLAB Function1/5(U1), MATLAB Function2/4(U1)
  MATLAB Function/1(X_ddot) -> X_ddot/1
  MATLAB Function2/1(Z_ddot) -> Z_ddot/1
  MATLAB Function1/1(Y_ddot) -> Y_ddot/1

== matlab function quad_dynamics/Complimentary_filter_phi/MATLAB Function ==
  data: X_ddot_in input; Phi output; Theta output; Y_ddot_in input; Z_ddot_in input
function [Phi, Theta] = Accels2Angles(X_ddot_in, Y_ddot_in,Z_ddot_in)
 

    % Calculate Roll (Phi) and Pitch (Theta) angles in radians
    Phi   = atan(-Y_ddot_in / Z_ddot_in);
    Theta = atan(-X_ddot_in / sqrt(Y_ddot_in^2 + Z_ddot_in^2));
end

== matlab function quad_dynamics/Oreintation ==
  data: angles input; q output
function q = euler_to_quat(angles)
    % Extract the Euler angles
    phi = angles(1);
    theta = angles(2);
    psi = angles(3);
    
    % Ferry's Euler to Quaternion Equations
    q0 = cos(phi/2)*cos(theta/2)*cos(psi/2) + sin(phi/2)*sin(theta/2)*sin(psi/2);
    q1 = sin(phi/2)*cos(theta/2)*cos(psi/2) - cos(phi/2)*sin(theta/2)*sin(psi/2);
    q2 = cos(phi/2)*sin(theta/2)*cos(psi/2) + sin(phi/2)*cos(theta/2)*sin(psi/2);
    q3 = cos(phi/2)*cos(theta/2)*sin(psi/2) - sin(phi/2)*sin(theta/2)*cos(psi/2);
    
    % Output as a 1-by-4 row vector (N-by-4 format)
    q = [q0, q1, q2, q3];
end

== matlab function quad_dynamics/Non linear Quadcopter plant/Rotational Dynamics/MATLAB Function ==
  data: phi_ddot output; theta_dot input; psi_dot input; Omega_r input; U2 input; Jr parameter; Ixx parameter; Iyy parameter; Izz parameter; l parameter
function phi_ddot = roll_acceleration( theta_dot, psi_dot, Omega_r, U2, Jr, Ixx, Iyy, Izz, l)


phi_ddot = (theta_dot * psi_dot * (Iyy - Izz) + Jr * theta_dot * Omega_r + l * U2) / Ixx;
end

== matlab function quad_dynamics/Non linear Quadcopter plant/Rotational Dynamics/MATLAB Function1 ==
  data: phi_dot input; theta_ddot output; psi_dot input; Omega_r input; U3 input; l parameter; Izz parameter; Iyy parameter; Ixx parameter; Jr parameter
function theta_ddot = pitch_acceleration(phi_dot, psi_dot, Omega_r, U3, l, Izz, Iyy, Ixx, Jr)


theta_ddot = (phi_dot * psi_dot * (Izz - Ixx) - Jr * phi_dot * Omega_r + l * U3) / Iyy;
end

== matlab function quad_dynamics/Non linear Quadcopter plant/Rotational Dynamics/MATLAB Function2 ==
  data: phi_dot input; psi_ddot output; theta_dot input; U4 input; Izz parameter; Iyy parameter; Ixx parameter
function psi_ddot = yaw_acceleration(phi_dot, theta_dot, U4, Izz, Iyy, Ixx)


psi_ddot = (theta_dot * phi_dot * (Ixx - Iyy) + U4) / Izz;
end

== matlab function quad_dynamics/Non linear Quadcopter plant/translation Dynamics/MATLAB Function ==
  data: phi input; X_ddot output; theta input; psi input; X_dot input; U1 input; Ax parameter; m parameter
function X_ddot = x_acceleration(phi, theta, psi, X_dot, U1, Ax, m)


X_ddot = ((sin(psi) * sin(phi) - cos(psi) * sin(theta) * cos(phi)) * U1 - Ax * X_dot) / m;
end

== matlab function quad_dynamics/Non linear Quadcopter plant/translation Dynamics/MATLAB Function1 ==
  data: phi input; Y_ddot output; theta input; psi input; Y_dot input; U1 input; Ay parameter; m parameter
function Y_ddot = y_acceleration(phi, theta, psi, Y_dot, U1, Ay, m)


Y_ddot = ((cos(psi) * sin(phi) + sin(psi) * sin(theta) * cos(phi)) * U1 - Ay * Y_dot) / m;
end

== matlab function quad_dynamics/Non linear Quadcopter plant/translation Dynamics/MATLAB Function2 ==
  data: phi input; Z_ddot output; theta input; Z_dot input; U1 input; Az parameter; g parameter; m parameter
function Z_ddot = z_acceleration(phi, theta, Z_dot, U1, Az, g, m)


Z_ddot = (m * g - (cos(theta) * cos(phi)) * U1 - Az * Z_dot) / m;
end

== matlab function quad_dynamics/Low level flight controller/Position control/MATLAB Function ==
  data: u_x input; phi_d output; u_y input; psi input; theta_d output
function [phi_d, theta_d] = compute_attitude_references(u_x, u_y, psi)
    % 1. Explicitly declare output sizes to satisfy the Simulink compiler
    phi_d   = 0.0; 
    theta_d = 0.0;

    g = 9.81;
    
    % 2. Rotation and transformation matrices
    R_psi = [cos(psi), -sin(psi);
             sin(psi),  cos(psi)];
         
    A_psi = R_psi * [0, 1; -1, 0];
    
    % 3. Process the control vector
    virtual_control = [u_x; u_y];
    Theta_hd = (-1 / g) * (A_psi \ virtual_control);
    
    % 4. Assign final values
    phi_d   = Theta_hd(1);
    theta_d = Theta_hd(2);
end

== matlab function quad_dynamics/Low level flight controller/MATLAB Function ==
  data: f_d input; tau_dx input; w1_sq output; w2_sq output; tau_dy input; w3_sq output; w4_sq output; tau_dz input
function [w1_sq, w2_sq, w3_sq, w4_sq] = Control_Allocation(f_d, tau_dx, tau_dy,tau_dz)
% MOTOR_MIXER Computes four rotor angular velocity squares from controller demands
% using structural constants from your initialization script.
%
% Inputs:
%   tau_dx   : Roll moment command (scalar, N-m)
%   tau_dy   : Pitch moment command (scalar, N-m)
%   tau_dz   : Yaw moment command (scalar, N-m)
%   f_d      : General vertical thrust command (scalar, N)
%
% Outputs:
%   w1_sq to w4_sq : Squared target angular speeds for motors 1 through 4 (rad/s)^2

    % =========================================================================
    % 1. ASSIGN QUADROTOR PARAMETERS (From your script)
    % =========================================================================
    % Converted parameters matching Sunny-sky A2212 / APC 10x4.5 dynamometer data:
    c_T = 1.3551e-05;   % Converted Thrust factor 'b' (N/(rad/s)^2)
    c_M = 2.6664e-07;   % Converted Drag/Torque factor 'd' (Nm/(rad/s)^2)
    arm_l = 0.2223;     % Distance from motor to center of mass 'l' (meters)

    % =========================================================================
    % 2. CONSTRUCT REFERENCE DEMAND VECTOR
    % =========================================================================
    % Scales your system inputs according to the row rules:
    control_vector = [ f_d / c_T;
                       tau_dx / (arm_l * c_T);
                       tau_dy / (arm_l * c_T);
                       tau_dz / c_M ];

    % =========================================================================
    % 3. CHASSIS ALLOCATION MATRIX (M4_dagger)
    % =========================================================================
    % Symmetric 45-degree structural pseudo-inverse matrix for X-configurations:
    M4_dagger = 0.25 * [ 1,  sqrt(2),  sqrt(2),  1;
                         1, -sqrt(2),  sqrt(2), -1;
                         1, -sqrt(2), -sqrt(2),  1;
                         1,  sqrt(2), -sqrt(2), -1 ];

    % =========================================================================
    % 4. COMPUTE SQUARED OUTPUTS
    % =========================================================================
    omega_squared = M4_dagger * control_vector;

    % Dynamic Guard: Enforce physical bounds (prevent negative speed squares)
    omega_squared = max(omega_squared, 0);

    % Map to separate output canvas ports
    w1_sq = omega_squared(1);
    w2_sq = omega_squared(2);
    w3_sq = omega_squared(3);
    w4_sq = omega_squared(4);
end

== matlab function quad_dynamics/Quadcopter plant/Rotational Dynamics/MATLAB Function1 ==
  data: phi_dot input; theta_ddot output; psi_dot input; Omega_r input; U3 input; l parameter; Izz parameter; Iyy parameter; Ixx parameter; Jr parameter
function theta_ddot = pitch_acceleration(phi_dot, psi_dot, Omega_r, U3, l, Izz, Iyy, Ixx, Jr)


theta_ddot = (phi_dot * psi_dot * (Izz - Ixx) - Jr * phi_dot * Omega_r + l * U3) / Iyy;
end

== matlab function quad_dynamics/Quadcopter plant/Rotational Dynamics/MATLAB Function ==
  data: phi_ddot output; theta_dot input; psi_dot input; Omega_r input; U2 input; Jr parameter; Ixx parameter; Iyy parameter; Izz parameter; l parameter
function phi_ddot = roll_acceleration( theta_dot, psi_dot, Omega_r, U2, Jr, Ixx, Iyy, Izz, l)


phi_ddot = (theta_dot * psi_dot * (Iyy - Izz) + Jr * theta_dot * Omega_r + l * U2) / Ixx;
end

== matlab function quad_dynamics/Quadcopter plant/Rotational Dynamics/MATLAB Function2 ==
  data: phi_dot input; psi_ddot output; theta_dot input; U4 input; Izz parameter; Iyy parameter; Ixx parameter
function psi_ddot = yaw_acceleration(phi_dot, theta_dot, U4, Izz, Iyy, Ixx)


psi_ddot = (theta_dot * phi_dot * (Ixx - Iyy) + U4) / Izz;
end

== matlab function quad_dynamics/Quadcopter plant/translation Dynamics/MATLAB Function ==
  data: phi input; X_ddot output; theta input; psi input; X_dot input; U1 input; Ax parameter; m parameter
function X_ddot = x_acceleration(phi, theta, psi, X_dot, U1, Ax, m)


X_ddot = ((sin(psi) * sin(phi) - cos(psi) * sin(theta) * cos(phi)) * U1 - Ax * X_dot) / m;
end

== matlab function quad_dynamics/Quadcopter plant/translation Dynamics/MATLAB Function1 ==
  data: phi input; Y_ddot output; theta input; psi input; Y_dot input; U1 input; Ay parameter; m parameter
function Y_ddot = y_acceleration(phi, theta, psi, Y_dot, U1, Ay, m)


Y_ddot = ((cos(psi) * sin(phi) + sin(psi) * sin(theta) * cos(phi)) * U1 - Ay * Y_dot) / m;
end

== matlab function quad_dynamics/Quadcopter plant/translation Dynamics/MATLAB Function2 ==
  data: phi input; Z_ddot output; theta input; Z_dot input; U1 input; Az parameter; g parameter; m parameter
function Z_ddot = z_acceleration(phi, theta, Z_dot, U1, Az, g, m)


Z_ddot = (m * g - (cos(theta) * cos(phi)) * U1 - Az * Z_dot) / m;
end
